simulink library "csbenchlab_sys"  (R2024a)
settings: Solver=VariableStepAuto  StartTime=0.0  StopTime=10.0  RelTol=1e-3
undefined symbols (not defined in the file or in its folder): extrinsic, LinearSystem_data, LinearSystem_DT, LinearSystem_params, LinearSystem_params_merged, LinearSystem_PT
settings Model: Creator=luka  LastModifiedBy=luka

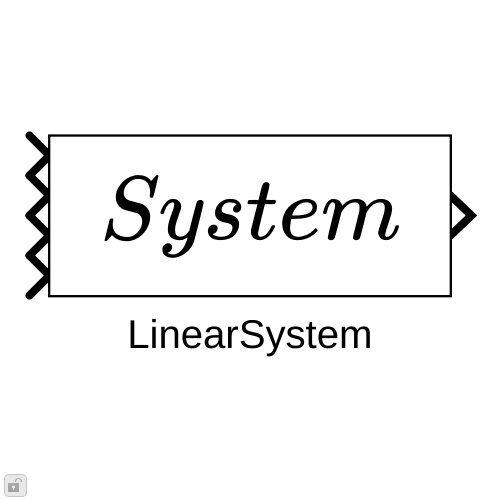
[thumbnail: Simulink's stored preview of the top-level diagram]
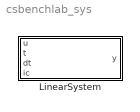
== system csbenchlab_sys ==
  LinearSystem : Subsystem  Tag=__cs_m_sys;  mask{params=LinearSystem_params, params_merged=LinearSystem_params_merged, data=LinearSystem_data, ParamsType=LinearSystem_PT, DataType=LinearSystem_DT, iid__=[0], pid__=[76 105 110 101 97 114 83 121 115 116 101 109 58 99 115 98 101 110 99 104 108 97 98]}
      mask prompts: params "Parameter struct:"

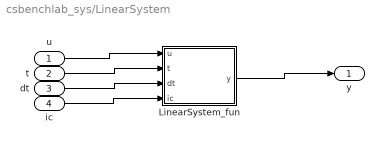
== system csbenchlab_sys/LinearSystem ==
  u : Inport
  t : Inport  Port=2
  dt : Inport  Port=3
  ic : Inport  Port=4
  LinearSystem_fun : MATLAB Function  TreatAsAtomicUnit=on
  y : Outport
  wires:
  u/1 -> LinearSystem_fun/1(u)
  t/1 -> LinearSystem_fun/2(t)
  dt/1 -> LinearSystem_fun/3(dt)
  ic/1 -> LinearSystem_fun/4(ic)
  LinearSystem_fun/1(y) -> y/1

== matlab function csbenchlab_sys/LinearSystem/LinearSystem_fun ==
  settings: updateMethod=DISCRETE
  data: u input; y output; t input; dt input; ic input; extrinsic parameter int32; iid__ parameter uint8; pid__ parameter uint8; data parameter DataType; params_merged parameter ParamsType
% __classname:="LinearSystem";
% __fnname:="fcn_bd7e311e9e354b488fdeb264b320d6ed";
% __input_args:="u, t, dt, ic, params_merged, data, pid__, iid__";
% __output_args:=" y";
% __ctor_args:="params_merged, 'Data', data, 'pid', pid__, 'iid', iid__";
% __cfg_args:=" ic";
% __step_args:="u, t, dt";
function y = fcn(u, t, dt, ic, extrinsic, iid__, pid__, data, params_merged)
  coder.extrinsic('fcn_bd7e311e9e354b488fdeb264b320d6ed_ext');
  if extrinsic
      y = zeros(size(ic));
      y = fcn_bd7e311e9e354b488fdeb264b320d6ed_ext(u, t, dt, ic, params_merged, data, pid__, iid__);
  else
      y = fcn_bd7e311e9e354b488fdeb264b320d6ed(u, t, dt, ic, params_merged, data, pid__, iid__);
  end
end

function y = fcn_bd7e311e9e354b488fdeb264b320d6ed(u, t, dt, ic, params_merged, data, pid__, iid__)
  persistent obj
  if isempty(obj)
    obj = LinearSystem(params_merged, 'Data', data, 'pid', pid__, 'iid', iid__);
    obj = obj.configure( ic);
  end
  [obj, y] = obj.step(u, t, dt);
end
